simulink model "step_response_01"  (R2024b)
settings: Solver=VariableStepAuto  StartTime=0.0  StopTime=10.0  RelTol=1e-3
values from neighbouring files (symbols this model uses):
  A = [0, 0, 0, 1, 0, 0 ... (first row only)    [parameter_init.m]
  B = [0, 0 ... (first row only)    [parameter_init.m]
  C = [1, 0, 0, 0, 0, 0 ... (first row only)    [parameter_init.m]
undefined symbols (not defined in the file or in its folder): K
settings Model: Creator=KevinNuo  LastModifiedBy=KevinNuo

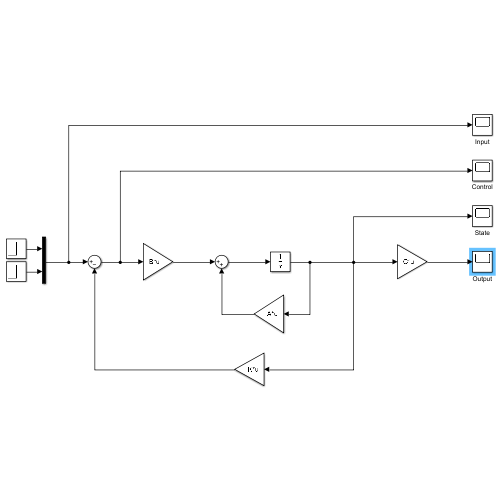
[thumbnail: Simulink's stored preview of the top-level diagram]
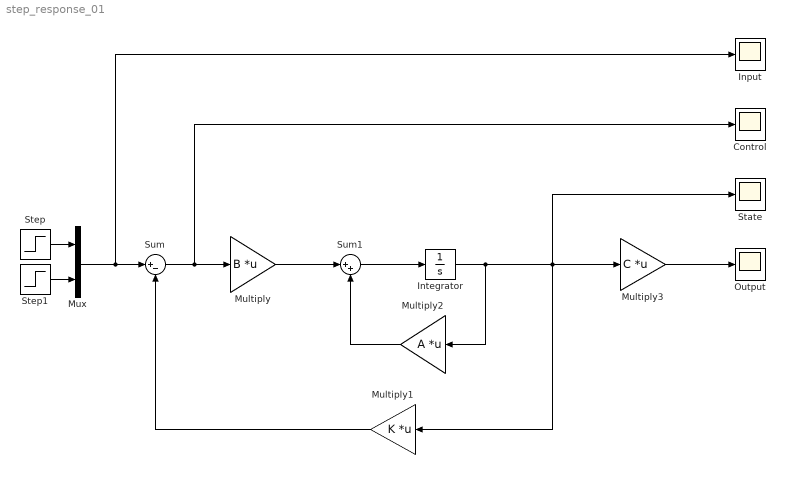
== system step_response_01 ==
  Control : Scope
  Input : Scope
  Integrator : Integrator
  Multiply : Gain  Gain=B  Multiplication=Matrix(K*u)
  Multiply1 : Gain  Gain=K  Multiplication=Matrix(K*u)
  Multiply2 : Gain  Gain=A  Multiplication=Matrix(K*u)
  Multiply3 : Gain  Gain=C  Multiplication=Matrix(K*u)
  Mux : Mux  Inputs=2
  Output : Scope
  State : Scope
  Step : Step  Time=0  After=0  SampleTime=0
  Step1 : Step  Time=0  SampleTime=0
  Sum : Sum  Inputs=|+-
  Sum1 : Sum  Inputs=|++
  wires:
  Step/1 -> Mux/1
  Step1/1 -> Mux/2
  Mux/1 -> Input/1, Sum/1
  Multiply1/1 -> Sum/2
  Sum/1 -> Control/1, Multiply/1
  Multiply/1 -> Sum1/1
  Sum1/1 -> Integrator/1
  Integrator/1 -> Multiply2/1, State/1, Multiply1/1, Multiply3/1
  Multiply2/1 -> Sum1/2
  Multiply3/1 -> Output/1
